simulink model "controle_malha_aberta"  (R2021a)
settings: Solver=VariableStepAuto  StartTime=0.0  StopTime=2.0  RelTol=1e-3
settings Model: Creator=caioc  LastModifiedBy=caioc

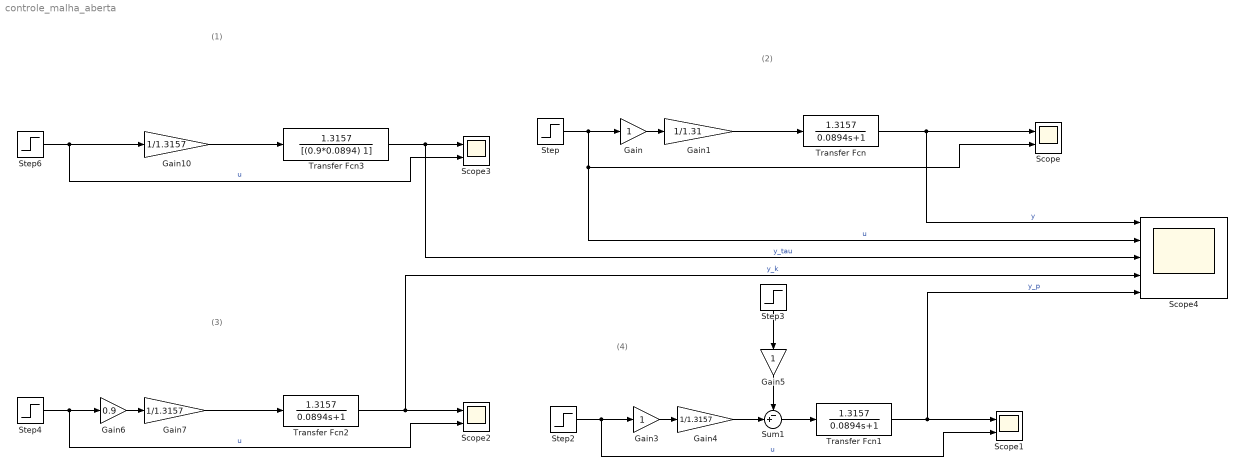
== system controle_malha_aberta ==
  note: (1)
  note: (2)
  note: (3)
  note: (4)
  Gain : Gain
  Gain1 : Gain  Gain=1/1.31
  Gain10 : Gain  Gain=1/1.3157
  Gain3 : Gain
  Gain4 : Gain  Gain=1/1.3157
  Gain5 : Gain
  Gain6 : Gain  Gain=0.9
  Gain7 : Gain  Gain=1/1.3157
  Scope{,1..3} (4 alike) : Scope  NumInputPorts=2
  Scope4 : Scope  NumInputPorts=5
  Step{,2,4,6} (4 alike) : Step  Time=0  After=10  SampleTime=0
  Step3 : Step  Time=0  After=0.45  SampleTime=0
  Sum1 : Sum  Inputs=-+|
  Transfer Fcn : TransferFcn  Numerator=[1.3157]  Denominator=[0.0894 1]
  Transfer Fcn1 : TransferFcn  Numerator=[1.3157]  Denominator=[0.0894 1]
  Transfer Fcn2 : TransferFcn  Numerator=[1.3157]  Denominator=[0.0894 1]
  Transfer Fcn3 : TransferFcn  Numerator=[1.3157]  Denominator=[(0.9*0.0894) 1]
  wires:
  Gain/1 -> Gain1/1
  Step/1 -> Scope4/2, Scope/2, Gain/1  "u"
  Transfer Fcn/1 -> Scope4/1, Scope/1  "y"
  Gain1/1 -> Transfer Fcn/1
  Gain3/1 -> Gain4/1
  Step2/1 -> Scope1/2, Gain3/1  "u"
  Sum1/1 -> Transfer Fcn1/1
  Gain4/1 -> Sum1/2
  Gain5/1 -> Sum1/1
  Transfer Fcn1/1 -> Scope1/1, Scope4/5  "y_p"
  Step3/1 -> Gain5/1
  Gain6/1 -> Gain7/1
  Step4/1 -> Scope2/2, Gain6/1  "u"
  Gain7/1 -> Transfer Fcn2/1
  Transfer Fcn2/1 -> Scope2/1, Scope4/4  "y_k"
  Step6/1 -> Gain10/1, Scope3/2  "u"
  Transfer Fcn3/1 -> Scope3/1, Scope4/3  "y_tau"
  Gain10/1 -> Transfer Fcn3/1
